simulink model "helicopter_MPC_moldovan"  (R2021b)
settings: Solver=ode45  StartTime=0.0  StopTime=T  RelTol=1e-3
InitFcn:
  | hwinit
values from neighbouring files (symbols this model uses):
  adingain = [1 1 1 1]    [matlab.mat]
  adinoffs = [0 0 0 0]    [matlab.mat]
  discrete_A = discrete_sys.A    [polish_MPC.m]
  discrete_B = discrete_sys.B    [polish_MPC.m]
  h = 0.01    [calibration.m]    (also in controller1.m; controller_LQR.m; controller_LQR_trajectory.m; controller_pole_EKF.m)
  P = [638567526.314  -8684287.96324  -748875.515442; -8684287.96324  5985173.52622  11443.8467884; -748875.515442  11443.8467884  886.337241088]    [matlab.mat]    (also in polish_MPC.m = P_inf)
  Q_MPC = [1000  0  0; 0  20  0; 0  0  0.1]    [matlab.mat]    (also in polish_MPC.m = [200000, 0, 0; 0, 40000, 0; 0, 0, 1000])
  R_MPC = 8    [matlab.mat]    (also in polish_MPC.m = [18])
  t_mpc = 0.2    [matlab.mat]    (also in polish_MPC.m = 0.01)
  ureeef = alpha_to_u(alpha_ref)    [polish_MPC.m]
  x_ref = [alpha_ref; alpha_dot_ref; omega_ref]    [controller1.m]    (also in controller_LQR.m = [alpha_ref; alpha_dot_ref; omega_ref]/0.9; controller_LQR_trajectory.m = [alpha_ref;alpha_dot_ref;omega_ref']; controller_pole_EKF.m; matlab.mat = [0.15 0 0])
  y_ref_desired = [0.15 0]    [matlab.mat]    (also in polish_MPC.m = [alpha_ref; omega_ref])
undefined symbols (not defined in the file or in its folder): HeliMexHandle
libraries: simulink x1, sharedTrackingLibrary x1, eeGeneralControl x1, mpclib x1, dspstat3 x1
settings Model: Creator=fkzhang  LastModifiedBy=lcaric
settings SolverCC: AlgebraicLoopSolver=TrustRegion
settings DataIOCC: LimitDataPoints=on  SaveFormat=Array  ReturnWorkspaceOutputs=off
settings OptimizationCC: BlockReduction=off  BooleanDataType=off  LifeSpan=inf
settings DebuggingCC: SaveWithParameterizedLinksMsg=none  UnderspecifiedInitializationDetection=Classic  MergeDetectMultiDrivingBlocksExec=none  SignalResolutionControl=TryResolveAllWithWarning  AllowSymbolicDim=off  SFUnexpectedBacktrackingDiag=warning  SFNoUnconditionalDefaultTransitionDiag=warning  SFExecutionAtInitializationDiag=none  SFMachineParentedDataDiag=warning  ArithmeticOperatorsInVariantConditions=warning
settings HardwareCC: ProdBitPerPointer=32  ProdBitPerSizeT=32  ProdBitPerPtrDiffT=32  ProdLargestAtomicFloat=None  ProdIntDivRoundTo=Undefined  ProdEndianess=Unspecified  ProdWordSize=32  ProdHWDeviceType=32-bit Generic  TargetBitPerPointer=64  TargetBitPerSizeT=64  TargetBitPerPtrDiffT=64  TargetLongLongMode=on  TargetIntDivRoundTo=Zero  TargetEndianess=LittleEndian  TargetWordSize=64  TargetHWDeviceType=MATLAB Host  ProdEqTarget=off
settings ModelReferenceCC: PropagateSignalLabelsOutOfModel=off
settings SFSimCC: SimUseLocalCustomCode=off  CustomCodeUndefinedFunction=UseInterfaceOnly
settings RTWCC: RTWUseLocalCustomCode=off
settings CodeAppCC: StateflowObjectComments=on
settings GRTTargetCC: TargetLangStandard=C89/C90 (ANSI)
settings ConfigComp: CovMetricSettings=dw  CovSaveCumulativeToWorkspaceVar=on  CovSaveSingleToWorkspaceVar=on  CovExternalEMLEnable=off  CovSFcnEnable=off

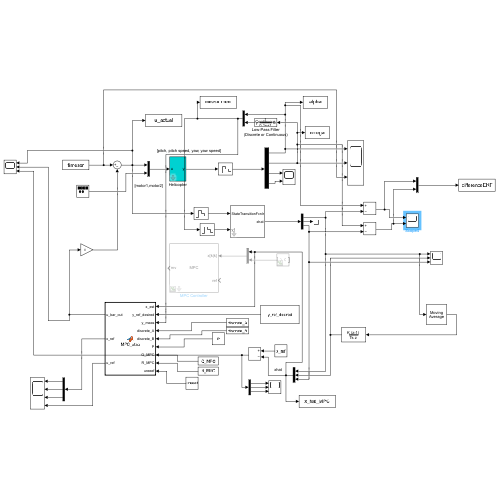
[thumbnail: Simulink's stored preview of the top-level diagram]
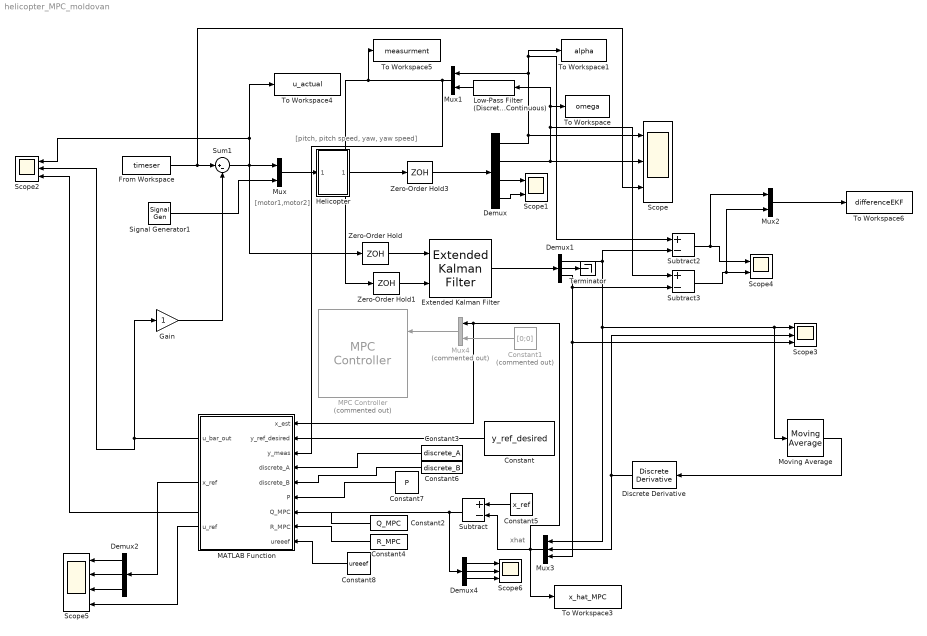
== system helicopter_MPC_moldovan ==
  note: xhat
  note: [pitch, pitch speed, yaw, yaw speed]
  note: [motor1,motor2]
  Constant : Constant  Value=y_ref_desired
  Constant1 : Constant  Commented=on  Value=[0;0]
  Constant2 : Constant  Value=Q_MPC
  Constant3 : Constant  Value=discrete_A
  Constant4 : Constant  Value=R_MPC
  Constant5 : Constant  Value=x_ref
  Constant6 : Constant  Value=discrete_B
  Constant7 : Constant  Value=P
  Constant8 : Constant  Value=ureeef
  Demux : Demux
  Demux1 : Demux  Outputs=3
  Demux2 : Demux  Outputs=3
  Demux4 : Demux  Outputs=3
  Discrete Derivative : simulink/Discrete/Discrete Derivative  gainval=1.0  ICPrevScaledInput=0.0  OutMin=[]  OutMax=[]  OutDataType=fixdt(1, 16)  OutScaling=2^-10  DoSatur=off
  Extended Kalman Filter : sharedTrackingLibrary/Extended Kalman Filter  StateTransitionFcn=nonlin_evolution  HasStateTransitionJacobianFcn=off  StateTransitionJacobianFcn=nonlin_jacobian  HasAdditiveProcessNoise=Additive  ProcessNoise=Q_kalman  HasTimeVaryingProcessNoise=off  HasStateTransitionFcnExtraArgument=1  InitialState=[0; 0; 0]  InitialStateCovariance=Q_kalman  MeasurementFcn1=nonlin_measurement_all  HasMeasurementJacobianFcn1=off  HasMeasurementEnablePort1=off  HasAdditiveMeasurementNoise1=Additive  MeasurementNoise1=R_kalman  HasTimeVaryingMeasurementNoise1=off  HasMeasurementFcnExtraArgument1=0  MeasurementFcn2=nonlin_measurement_omega  HasMeasurementJacobianFcn2=off  HasMeasurementEnablePort2=off  HasAdditiveMeasurementNoise2=Additive  MeasurementNoise2=10  HasTimeVaryingMeasurementNoise2=off  HasMeasurementFcnExtraArgument2=0  MeasurementFcn3=myMeasurementFcn  HasMeasurementJacobianFcn3=off  HasMeasurementEnablePort3=off  HasAdditiveMeasurementNoise3=Additive  MeasurementNoise3=1  HasTimeVaryingMeasurementNoise3=off  HasMeasurementFcnExtraArgument3=0  MeasurementFcn4=myMeasurementFcn  HasMeasurementJacobianFcn4=off  HasMeasurementEnablePort4=off  HasAdditiveMeasurementNoise4=Additive  MeasurementNoise4=1  HasTimeVaryingMeasurementNoise4=off  HasMeasurementFcnExtraArgument4=0  MeasurementFcn5=myMeasurementFcn  HasMeasurementJacobianFcn5=off  HasMeasurementEnablePort5=off  HasAdditiveMeasurementNoise5=Additive  MeasurementNoise5=1  HasTimeVaryingMeasurementNoise5=off  HasMeasurementFcnExtraArgument5=0  EnableMultirate=off  StateTransitionFcnSampleTime=1  MeasurementFcn1SampleTime=1  MeasurementFcn2SampleTime=1  MeasurementFcn3SampleTime=1  MeasurementFcn4SampleTime=1  MeasurementFcn5SampleTime=1  UseCurrentEstimator=on  OutputStateCovariance=off  DataType=double  SampleTime=0.02  NumberOfMeasurements=1
      settings: SourceProductBaseCode=AE,PW,CT,DR,TF,ID,LP,NV,AR,RO,RR,UV,VE
  From Workspace : FromWorkspace  VariableName=timeser
  Gain : Gain
  Helicopter : Subsystem  mask{Ts=h}
      mask prompts: Ts "sampletime"
      mask init:
      | sf_heli_init
      mask Display:
      | port_label('input',1,'u');
      | port_label('output',1,'y');
  Low-Pass Filter (Discrete or Continuous) : eeGeneralControl/Low-Pass Filter (Discrete or Continuous)  K=1  T=0.1  B=inf  A=-inf  init_option=Inherited from block input  x0=0  Ts=0
  MATLAB Function : MATLAB Function  TreatAsAtomicUnit=on  SystemSampleTime=t_mpc
  MPC Controller : mpclib/MPC Controller  Commented=on  SCDEnableBlockLinearizationSpecification=on  mpcobj=mpcobj  x0=state  is_multiple=0  enable_value=0  return_u0=off  updateMPCinCallerWorkspace=on  md_inport=off  mv_inport=off  uref_inport=off  return_cost=off  return_mvseq=off  return_qpstatus=off  return_xseq=off  return_state=off  return_ovseq=off  state_inport=on  umin_inport=off  umax_inport=off  ymin_inport=off  ymax_inport=off  cc_inport=off  ywt_inport=off  uwt_inport=off  duwt_inport=off  rhoeps_inport=off  pm_inport=off  MaximumP=10  HorizonChoice=FixedHorizon  n_ts=0.01  n_p=500  n_mv=1  n_md=0  n_ud=0  n_mo=2  n_uo=0  BlockDataType=double  SampleTimeInherited=off  switch_inport=off
  Moving Average : dspstat3/Moving Average  Method=Sliding window  ForgettingFactorPort=off  SpecifyWindowLength=on  WindowLength=5  ForgettingFactor=0.9  SimulateUsing=Code generation
  Mux : Mux  Inputs=2
  Mux1 : Mux  Inputs=2
  Mux2 : Mux  Inputs=2
  Mux3 : Mux  Inputs=3
  Mux4 : Mux  Commented=on  Inputs=2
  Scope{,2..3,6} (4 alike) : Scope  NumInputPorts=3
  Scope1 : Scope  NumInputPorts=2
  Scope4 : Scope  NumInputPorts=2
  Scope5 : Scope  NumInputPorts=4
  Signal Generator1 : SignalGenerator  WaveForm=square  Amplitude=0  Frequency=1/20
  Subtract : Sum  Inputs=+-
  Subtract2 : Sum  Inputs=+-
  Subtract3 : Sum  Inputs=+-
  Sum1 : Sum  Inputs=|+-
  Terminator : Terminator
  To Workspace : ToWorkspace  VariableName=omega  SaveFormat=Timeseries  SampleTime=-1
  To Workspace1 : ToWorkspace  VariableName=alpha  SaveFormat=Timeseries  SampleTime=-1
  To Workspace3 : ToWorkspace  VariableName=x_hat_MPC  SaveFormat=Timeseries  SampleTime=-1
  To Workspace4 : ToWorkspace  VariableName=u_actual  SaveFormat=Timeseries  SampleTime=-1
  To Workspace5 : ToWorkspace  VariableName=measurment  SaveFormat=Timeseries  SampleTime=-1
  To Workspace6 : ToWorkspace  VariableName=differenceEKF  SaveFormat=Timeseries  SampleTime=-1
  Zero-Order Hold : ZeroOrderHold  SampleTime=0.02
  Zero-Order Hold1 : ZeroOrderHold  SampleTime=0.02
  Zero-Order Hold3 : ZeroOrderHold  SampleTime=0.05
  wires:
  Mux/1 -> Helicopter/1(In1)
  Signal Generator1/1 -> Mux/2
  Demux/2 -> Low-Pass Filter (Discrete or Continuous)/1, To Workspace/1, Subtract3/1, Scope/2
  Demux/3 -> Scope1/1
  Demux/4 -> Scope1/2
  From Workspace/1 -> Sum1/1, Scope/3
  Demux/1 -> Subtract2/1, To Workspace1/1, Mux1/1, Scope/1
  Mux1/1 -> To Workspace5/1, Zero-Order Hold1/1, MATLAB Function/3(y_meas)
  Helicopter/1(Out1) -> Zero-Order Hold3/1
  Sum1/1 -> To Workspace4/1, Scope2/1, Zero-Order Hold/1, Mux/1
  Subtract/1 -> Scope2/3, Demux4/1
  Constant5/1 -> Subtract/1
  Zero-Order Hold/1 -> Extended Kalman Filter/1
  Zero-Order Hold1/1 -> Extended Kalman Filter/2
  Extended Kalman Filter/1 -> Demux1/1
  Demux1/3 -> Subtract3/2, Mux3/3, Scope3/3
  Subtract2/1 -> Mux2/1, Scope4/1
  Subtract3/1 -> Mux2/2, Scope4/2
  Mux2/1 -> To Workspace6/1
  Low-Pass Filter (Discrete or Continuous)/1 -> Mux1/2
  Demux1/1 -> Subtract2/2, Mux3/1, Moving Average/1, Scope3/1
  Discrete Derivative/1 -> Scope3/2, Mux3/2
  Mux3/1 -> MATLAB Function/1(x_est), Mux4/1, To Workspace3/1, Subtract/2
  Moving Average/1 -> Discrete Derivative/1
  Demux1/2 -> Terminator/1
  Demux4/1 -> Scope6/1
  Demux4/3 -> Scope6/3
  Demux4/2 -> Scope6/2
  Constant/1 -> MATLAB Function/2(y_ref_desired)
  Mux4/1 -> MPC Controller/1
  Constant1/1 -> Mux4/2
  Constant7/1 -> MATLAB Function/6(P)
  Constant6/1 -> MATLAB Function/5(discrete_B)
  Constant3/1 -> MATLAB Function/4(discrete_A)
  MATLAB Function/1(u_bar_out) -> Gain/1, Scope2/2
  Zero-Order Hold3/1 -> Demux/1
  Constant2/1 -> MATLAB Function/7(Q_MPC)
  Constant4/1 -> MATLAB Function/8(R_MPC)
  MATLAB Function/2(x_ref) -> Demux2/1
  MATLAB Function/3(u_ref) -> Scope5/4
  Demux2/1 -> Scope5/1
  Demux2/2 -> Scope5/2
  Demux2/3 -> Scope5/3
  Constant8/1 -> MATLAB Function/9(ureeef)
  Gain/1 -> Sum1/2

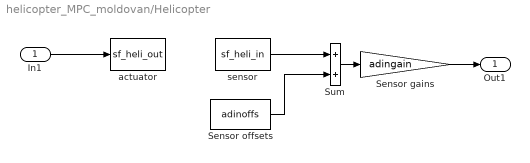
== system helicopter_MPC_moldovan/Helicopter ==
  In1 : Inport
  Sensor gains : Gain  Gain=adingain
  Sensor offsets : Constant  Value=adinoffs
  Sum : Sum
  actuator : M-S-Function  FunctionName=sf_heli_out  Parameters=HeliMexHandle,Ts
  sensor : M-S-Function  FunctionName=sf_heli_in  Parameters=HeliMexHandle
  Out1 : Outport  VectorParamsAs1DForOutWhenUnconnected=off
  wires:
  sensor/1 -> Sum/1
  In1/1 -> actuator/1
  Sensor offsets/1 -> Sum/2
  Sum/1 -> Sensor gains/1
  Sensor gains/1 -> Out1/1

== matlab function helicopter_MPC_moldovan/MATLAB Function ==
  data: x_est input; u_bar_out output; y_ref_desired input; y_meas input; discrete_A input; discrete_B input; P input; Q_MPC input; R_MPC input; x_ref output; u_ref output; ureeef input
function [u_bar_out, x_ref, u_ref] = MPC_step(x_est, y_ref_desired, y_meas, discrete_A, discrete_B, P, Q_MPC, R_MPC, ureeef)
    n_y = 2;
    n_x = 3;
    n_u =1;

    %Q_MPC = [2000, 0, 0; 0, 20, 0; 0, 0, 10];
    %R_MPC = [5];


  
    C = [1, 0, 0; 0, 0, 1];
    
    % Constraints
    x_min = [-pi/4; -3; -335];
    x_max = [ pi/4;  3; 337];
    u_lb = [-1];
    u_ub = [1];

    
    rho = 100000;
    N = 150; % 3sec


    u_bar = zeros(1, N);

    d_hat = zeros(n_y,1);
    d_hat(1:2) = y_meas(1:2) - C(1:2,:) * x_est;


    %discrete_sys = c2d(ss(A_lin,B_lin,C,0,0.1));

    %[x_ref, u_ref] = optimal_target_selectionKALMAN(discrete_A, discrete_B, C, [1], y_ref_desired, d_hat, u_lb, u_ub, x_min, x_max, Q_MPC);
    
    x_ref = [y_ref_desired(1);0; y_ref_desired(2)];
    u_ref = [ureeef];

    [x_bar, u_bar] = solve_offset_free_mpc(discrete_A, discrete_B, Q_MPC, R_MPC, P, x_est, N, u_lb, u_ub, x_ref, u_ref, x_min, x_max, rho);

    u_bar_out = u_bar(1, 1);

end

% function [x_ref_opt, u_ref_opt] = optimal_target_selectionKALMAN(A, B, C, R, y_ref, d_hat, u_lb, u_ub, x_min, x_max)
%     n_x = size(A,1);
%     n_u = size(B,2);
% 
%     x_ref = sdpvar(n_x, 1);
%     u_ref = sdpvar(n_u, 1);
% 
%     constraints = [];
%     constraints = [constraints, (eye(n_x) - A) * x_ref == B * u_ref];
%     constraints = [constraints, C * x_ref + d_hat == y_ref];
%     constraints = [constraints, u_lb <= u_ref <= u_ub];
%     constraints = [constraints, x_min <= x_ref <= x_max];
% 
%     objective = u_ref' * eye(n_u) * u_ref;
% 
%     opts = sdpsettings('solver','quadprog','verbose',0);
%     optimize(constraints, objective, opts);
% 
%     x_ref_opt = value(x_ref);
%     u_ref_opt = value(u_ref);
% end
